simulink model "chap5_2sim"  (Simulink 3.00)
settings: Solver=ode4  StartTime=0.0  StopTime=1.0  RelTol=1e-3
settings Model: SaveTime=off  SaveOutput=off  Decimation=100  LastModifiedBy=liu

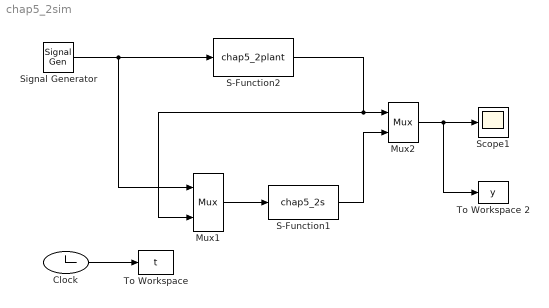
== system chap5_2sim ==
  Clock : Clock
  Mux1 : Mux  Inputs=2
      settings: DisplayOption=none
  Mux2 : Mux  Inputs=2
      settings: DisplayOption=none
  S-Function1 : S-Function  FunctionName=chap5_2s  PortCounts=[]  SFunctionModules=''
  S-Function2 : S-Function  FunctionName=chap5_2plant  PortCounts=[]  SFunctionModules=''
  Scope1 : Scope
      settings: TimeRange=0.2  YMin=-0.25  YMax=3  SaveToWorkspace=off  SaveName=ScopeData  MaxRows=50000  Decimation=0.001  SampleInput=on  SampleTime=0.001
  Signal Generator : SignalGenerator  WaveForm=sine  Amplitude=0.5  Frequency=3  Units=Hertz
  To Workspace : ToWorkspace  VariableName=t  SampleTime=-1  SaveFormat=Matrix
  To Workspace 2 : ToWorkspace  VariableName=y  SampleTime=-1  SaveFormat=Matrix
  wires:
  Mux1/1 -> S-Function1/1
  S-Function2/1 -> Mux1/2, Mux2/1
  Signal Generator/1 -> S-Function2/1, Mux1/1
  S-Function1/1 -> Mux2/2
  Clock/1 -> To Workspace/1
  Mux2/1 -> Scope1/1, To Workspace 2/1
